simulink model "Motoring_Gear"  (R2024a)
settings: Solver=VariableStepAuto  StartTime=0.0  StopTime=2  FixedStep=1e-6  MaxStep=1e-6  RelTol=1e-6
values from neighbouring files (symbols this model uses):
  B_mod = 0    [Motoring_Gear_param.m]
  Bdc = 1e-4    (= 0.0001)    [Motoring_Gear_param.m]
  BL = 5    [Motoring_Gear_param.m]
  Bs = 1e10    (= 10000000000)    [Motoring_Gear_param.m]
  Bsn = 0    [Motoring_Gear_param.m]
  flux = 0.0563    [Motoring_Gear_param.m]
  J_mod = 5.71e-4    (= 0.000571)    [Motoring_Gear_param.m]
  Jdc = 0.0003    [Motoring_Gear_param.m]
  Jsn = 3.16e-4    (= 0.000316)    [Motoring_Gear_param.m]
  Kag = 0.001    [Motoring_Gear_param.m]
  Kc = 1000000    [Motoring_Gear_param.m]
  Ke = 0.0164    [Motoring_Gear_param.m]
  Kt = 0.0164    [Motoring_Gear_param.m]
  Ld = 3e-5    (= 3e-05)    [Motoring_Gear_param.m]
  Ldc = 8.76e-5    (= 8.76e-05)    [Motoring_Gear_param.m]
  Lq = 3e-5    (= 3e-05)    [Motoring_Gear_param.m]
  Pa = 2    [Motoring_Gear_param.m]
  Psn = 9    [Motoring_Gear_param.m]
  q_mod = 11    [Motoring_Gear_param.m]
  Rs = 0.01    [Motoring_Gear_param.m]
  Rs_dc = 0.01    [Motoring_Gear_param.m]
  velocity_Ki_pi = Bdc*motor_bw    (= 0.0628318530718)    [Motoring_Gear_param.m]
  velocity_Kp_pi = Jdc*motor_bw    (= 0.188495559215)    [Motoring_Gear_param.m]
libraries: cstblocks x2
(part 1 of 2)
settings Model: Creator=User  LastModifiedBy=edlin
settings DebuggingCC: UnconnectedInputMsg=warning  UnconnectedOutputMsg=warning  UnconnectedLineMsg=warning
settings ModelReferenceCC: EnableRefExpFcnMdlSchedulingChecks=on
settings RTWCC: GPUComputeCapability=3.5  DLArmComputeVersion=19.05

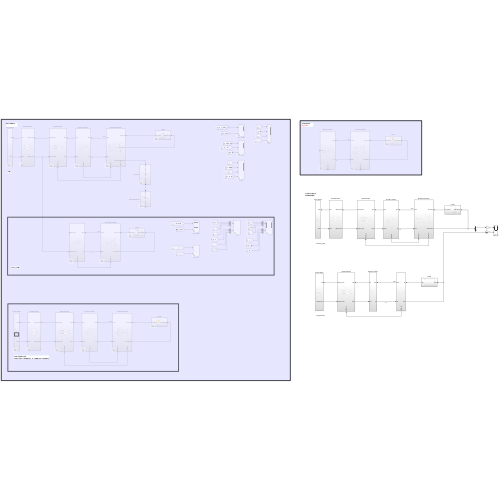
[thumbnail: Simulink's stored preview of the top-level diagram]
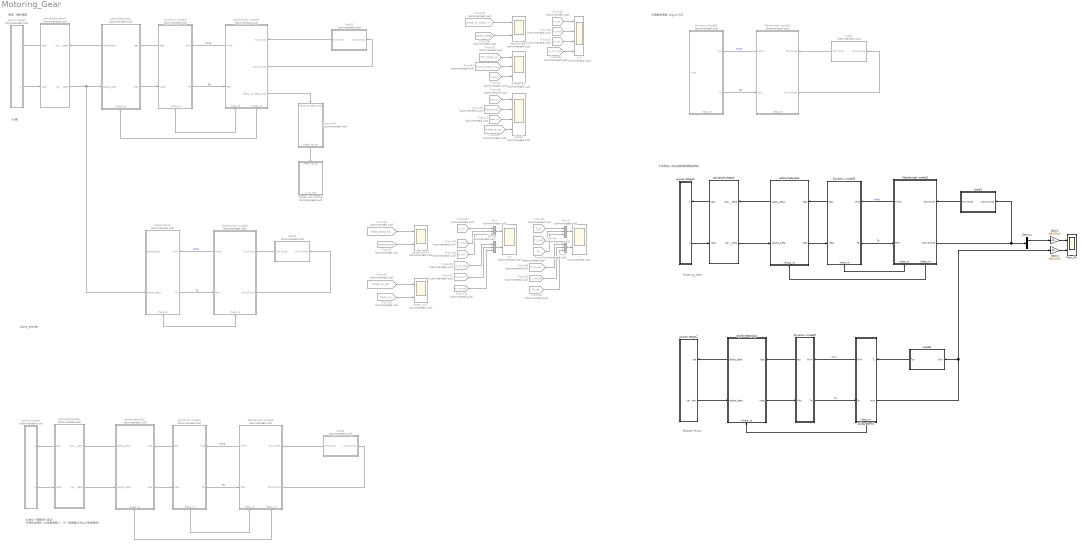
== system Motoring_Gear ==
  note: dq軸=>電壓源打直流
      | 中環或內還其一加負載當輸入，另一個當輸出(BL=0無負載角)
  note: Alpha_beta軸
  note: dq軸
  note: 反電動勢模擬 Kag=0.001
  note: 轉速、轉矩模擬
  note: 步進馬達vs磁性齒輪電機轉速模擬
  note: Motoring_Gear
  note: Stepper Motor
  Demux : Demux  Outputs=2
  Dynamic model1 : Subsystem  Commented=on
      settings: PortSchema="{\"entries\":[{\"content\":{\"sides\":[{\"content\":{\"connectorIds\":[\"In1\"]},\"type\":\"ConnectorPlacement.EquallySpacedRectSide\",\"uuid\":\"7c4d09e5-7ce3-4b20-8435-0def56d6c449\"},{\"content\":{\"connectorIds\":[\"In2\",\"Out1\"],\"side\":\"RIGHT\"},\"type\":\"ConnectorPlacement.EquallySpacedRectSide\",\"uuid\":\"93c63514-3f6b-48a8-aca2-b188521502f4\"},{\"content\":{\"connectorIds\":[],\"side\":\"TOP\"},\"type\":\"ConnectorPlacement.EquallySpacedRectSide\",\"uuid\":\"471dc423-a39c-4f8b-97d0-231d7e49bf1b\"},{\"content\":{\"connectorIds\":[\"Out2\"],\"side\":\"BOTTOM\"},\"type\":\"ConnectorPlacement.EquallySpacedRectSide\",\"uuid\":\"925e2c8f-0b09-4674-959a-18ac97fd648f\"}]},\"type\":\"ConnectorPlacement.EquallySpacedConnector\",\"uuid\":\"0274136e-6574-4791-859e-bbd37aa1b7b6\"}],\"packageUris\":[\"http://schema.mathworks.com/mf0/Connector/R2020b\"],\"version\":\"1.0\"}"
  Dynamic model2 : Subsystem
      settings: PortSchema="{\"entries\":[{\"content\":{\"sides\":[{\"content\":{\"connectorIds\":[\"Out3\",\"In1\"]},\"type\":\"ConnectorPlacement.EquallySpacedRectSide\",\"uuid\":\"7c4d09e5-7ce3-4b20-8435-0def56d6c449\"},{\"content\":{\"connectorIds\":[\"In2\",\"Out1\"],\"side\":\"RIGHT\"},\"type\":\"ConnectorPlacement.EquallySpacedRectSide\",\"uuid\":\"93c63514-3f6b-48a8-aca2-b188521502f4\"},{\"content\":{\"connectorIds\":[],\"side\":\"TOP\"},\"type\":\"ConnectorPlacement.EquallySpacedRectSide\",\"uuid\":\"471dc423-a39c-4f8b-97d0-231d7e49bf1b\"},{\"content\":{\"connectorIds\":[\"Out2\"],\"side\":\"BOTTOM\"},\"type\":\"ConnectorPlacement.EquallySpacedRectSide\",\"uuid\":\"925e2c8f-0b09-4674-959a-18ac97fd648f\"}]},\"type\":\"ConnectorPlacement.EquallySpacedConnector\",\"uuid\":\"0274136e-6574-4791-859e-bbd37aa1b7b6\"}],\"packageUris\":[\"http://schema.mathworks.com/mf0/Connector/R2020b\"],\"version\":\"1.0\"}"
  Dynamic model3 : Subsystem  Commented=on
      settings: PortSchema="{\"entries\":[{\"content\":{\"sides\":[{\"content\":{\"connectorIds\":[\"Out3\",\"In1\"]},\"type\":\"ConnectorPlacement.EquallySpacedRectSide\",\"uuid\":\"7c4d09e5-7ce3-4b20-8435-0def56d6c449\"},{\"content\":{\"connectorIds\":[\"In2\",\"Out1\"],\"side\":\"RIGHT\"},\"type\":\"ConnectorPlacement.EquallySpacedRectSide\",\"uuid\":\"93c63514-3f6b-48a8-aca2-b188521502f4\"},{\"content\":{\"connectorIds\":[],\"side\":\"TOP\"},\"type\":\"ConnectorPlacement.EquallySpacedRectSide\",\"uuid\":\"471dc423-a39c-4f8b-97d0-231d7e49bf1b\"},{\"content\":{\"connectorIds\":[\"Out2\"],\"side\":\"BOTTOM\"},\"type\":\"ConnectorPlacement.EquallySpacedRectSide\",\"uuid\":\"925e2c8f-0b09-4674-959a-18ac97fd648f\"}]},\"type\":\"ConnectorPlacement.EquallySpacedConnector\",\"uuid\":\"0274136e-6574-4791-859e-bbd37aa1b7b6\"}],\"packageUris\":[\"http://schema.mathworks.com/mf0/Connector/R2020b\"],\"version\":\"1.0\"}"
  Dynamic model4 : Subsystem  Commented=on
      settings: PortSchema="{\"entries\":[{\"content\":{\"sides\":[{\"content\":{\"connectorIds\":[\"Out3\",\"In1\"]},\"type\":\"ConnectorPlacement.EquallySpacedRectSide\",\"uuid\":\"7c4d09e5-7ce3-4b20-8435-0def56d6c449\"},{\"content\":{\"connectorIds\":[\"In2\",\"Out1\"],\"side\":\"RIGHT\"},\"type\":\"ConnectorPlacement.EquallySpacedRectSide\",\"uuid\":\"93c63514-3f6b-48a8-aca2-b188521502f4\"},{\"content\":{\"connectorIds\":[],\"side\":\"TOP\"},\"type\":\"ConnectorPlacement.EquallySpacedRectSide\",\"uuid\":\"471dc423-a39c-4f8b-97d0-231d7e49bf1b\"},{\"content\":{\"connectorIds\":[\"Out2\"],\"side\":\"BOTTOM\"},\"type\":\"ConnectorPlacement.EquallySpacedRectSide\",\"uuid\":\"925e2c8f-0b09-4674-959a-18ac97fd648f\"}]},\"type\":\"ConnectorPlacement.EquallySpacedConnector\",\"uuid\":\"0274136e-6574-4791-859e-bbd37aa1b7b6\"}],\"packageUris\":[\"http://schema.mathworks.com/mf0/Connector/R2020b\"],\"version\":\"1.0\"}"
  Dynamic model7 : Subsystem
      settings: PortSchema="{\"entries\":[{\"content\":{\"sides\":[{\"content\":{\"connectorIds\":[\"Out2\",\"In1\"]},\"type\":\"ConnectorPlacement.EquallySpacedRectSide\",\"uuid\":\"2f3a701f-5eea-44d1-b3a7-dbc1fa0e5c0a\"},{\"content\":{\"connectorIds\":[\"In2\",\"Out1\"],\"side\":\"RIGHT\"},\"type\":\"ConnectorPlacement.EquallySpacedRectSide\",\"uuid\":\"f1e2848b-d963-4e60-9d2d-973e23e5c5d3\"},{\"content\":{\"connectorIds\":[],\"side\":\"TOP\"},\"type\":\"ConnectorPlacement.EquallySpacedRectSide\",\"uuid\":\"f63106b5-8217-4120-80d6-773e81ca5be0\"}]},\"type\":\"ConnectorPlacement.EquallySpacedConnector\",\"uuid\":\"f5c5420c-1a40-42b7-b8dc-8ae6d2428c7a\"}],\"packageUris\":[\"http://schema.mathworks.com/mf0/Connector/R2020b\"],\"version\":\"1.0\"}"
  From25 : From  Commented=on  GotoTag=theta_re_theta_rm
  From26 : From  Commented=on  GotoTag=delta_theta  TagVisibility=global
  From27 : From  Commented=on  GotoTag=theta_rm  TagVisibility=global
  From28 : From  Commented=on  GotoTag=w_rm_res  TagVisibility=global
  From29 : From  Commented=on  GotoTag=theta_re_res  TagVisibility=global
  From30 : From  Commented=on  GotoTag=delta_theta_ab  TagVisibility=global
  From31 : From  Commented=on  GotoTag=delta_theta  TagVisibility=global
  From32 : From  Commented=on  GotoTag=theta_rm_ab  TagVisibility=global
  From33 : From  Commented=on  GotoTag=theta_rm  TagVisibility=global
  From34 : From  Commented=on  GotoTag=w_sn_ab  TagVisibility=global
  From35 : From  Commented=on  GotoTag=w_sn  TagVisibility=global
  From36 : From  Commented=on  GotoTag=w_mod  TagVisibility=global
  From37 : From  Commented=on  GotoTag=Psn_theta_sn  TagVisibility=global
  From38 : From  Commented=on  GotoTag=w_rm  TagVisibility=global
  From39 : From  Commented=on  GotoTag=T_sn_ab  TagVisibility=global
  From40 : From  Commented=on  GotoTag=T_sn  TagVisibility=global
  From41 : From  Commented=on  GotoTag=T_mod  TagVisibility=global
  From42 : From  Commented=on  GotoTag=Te  TagVisibility=global
  From43 : From  Commented=on  GotoTag=Pmod_theta_mod  TagVisibility=global
  From44 : From  Commented=on  GotoTag=theta_re  TagVisibility=global
  From45 : From  Commented=on  GotoTag=w_sn  TagVisibility=global
  From46 : From  Commented=on  GotoTag=w_mod  TagVisibility=global
  From47 : From  Commented=on  GotoTag=w_rm  TagVisibility=global
  From48 : From  Commented=on  GotoTag=theta_sn  TagVisibility=global
  From49 : From  Commented=on  GotoTag=theta_mod  TagVisibility=global
  From50 : From  Commented=on  GotoTag=w_rm_ab  TagVisibility=global
  From51 : From  Commented=on  GotoTag=w_mod_ab  TagVisibility=global
  From52 : From  Commented=on  GotoTag=Te_ab  TagVisibility=global
  From53 : From  Commented=on  GotoTag=T_mod_ab  TagVisibility=global
  Gain1 : Gain  Gain=60/(2*pi)
  Gain4 : Gain  Gain=60/(2*pi)
  Load1 : Subsystem  Commented=on
  Load2 : Subsystem
  Load3 : Subsystem  Commented=on
  Load4 : Subsystem  Commented=on
  Load5 : Subsystem  Commented=on
  Load6 : Subsystem
  Mechanical model1 : Subsystem  Commented=on
      settings: PortSchema="{\"entries\":[{\"content\":{\"sides\":[{\"content\":{\"connectorIds\":[\"Out2\",\"In1\"]},\"type\":\"ConnectorPlacement.EquallySpacedRectSide\",\"uuid\":\"27605504-0523-4623-b6f6-c9db4039f2d5\"},{\"content\":{\"connectorIds\":[\"In3\",\"Out1\"],\"side\":\"RIGHT\"},\"type\":\"ConnectorPlacement.EquallySpacedRectSide\",\"uuid\":\"20e727a9-aae7-4835-9463-ae6805ad2222\"},{\"content\":{\"connectorIds\":[],\"side\":\"TOP\"},\"type\":\"ConnectorPlacement.EquallySpacedRectSide\",\"uuid\":\"646511f2-a7bf-4324-af53-134f9ba550e9\"},{\"content\":{\"connectorIds\":[\"In2\"],\"side\":\"BOTTOM\"},\"type\":\"ConnectorPlacement.EquallySpacedRectSide\",\"uuid\":\"7eed8b1f-570c-458f-9984-581d7b55b244\"}]},\"type\":\"ConnectorPlacement.EquallySpacedConnector\",\"uuid\":\"62067768-bb43-41b2-88f6-4544d79748ee\"}],\"packageUris\":[\"http://schema.mathworks.com/mf0/Connector/R2020b\"],\"version\":\"1.0\"}"
  Mechanical model2 : Subsystem
      settings: PortSchema="{\"entries\":[{\"content\":{\"sides\":[{\"content\":{\"connectorIds\":[\"Out3\",\"In1\"]},\"type\":\"ConnectorPlacement.EquallySpacedRectSide\",\"uuid\":\"27605504-0523-4623-b6f6-c9db4039f2d5\"},{\"content\":{\"connectorIds\":[\"In3\",\"Out1\"],\"side\":\"RIGHT\"},\"type\":\"ConnectorPlacement.EquallySpacedRectSide\",\"uuid\":\"20e727a9-aae7-4835-9463-ae6805ad2222\"},{\"content\":{\"connectorIds\":[],\"side\":\"TOP\"},\"type\":\"ConnectorPlacement.EquallySpacedRectSide\",\"uuid\":\"646511f2-a7bf-4324-af53-134f9ba550e9\"},{\"content\":{\"connectorIds\":[\"In2\",\"Out2\"],\"side\":\"BOTTOM\"},\"type\":\"ConnectorPlacement.EquallySpacedRectSide\",\"uuid\":\"7eed8b1f-570c-458f-9984-581d7b55b244\"}]},\"type\":\"ConnectorPlacement.EquallySpacedConnector\",\"uuid\":\"62067768-bb43-41b2-88f6-4544d79748ee\"}],\"packageUris\":[\"http://schema.mathworks.com/mf0/Connector/R2020b\"],\"version\":\"1.0\"}"
  Mechanical model4 : Subsystem  Commented=on
      settings: PortSchema="{\"entries\":[{\"content\":{\"sides\":[{\"content\":{\"connectorIds\":[\"Out3\",\"In1\"]},\"type\":\"ConnectorPlacement.EquallySpacedRectSide\",\"uuid\":\"27605504-0523-4623-b6f6-c9db4039f2d5\"},{\"content\":{\"connectorIds\":[\"In3\",\"Out1\"],\"side\":\"RIGHT\"},\"type\":\"ConnectorPlacement.EquallySpacedRectSide\",\"uuid\":\"20e727a9-aae7-4835-9463-ae6805ad2222\"},{\"content\":{\"connectorIds\":[],\"side\":\"TOP\"},\"type\":\"ConnectorPlacement.EquallySpacedRectSide\",\"uuid\":\"646511f2-a7bf-4324-af53-134f9ba550e9\"},{\"content\":{\"connectorIds\":[\"In2\",\"Out2\"],\"side\":\"BOTTOM\"},\"type\":\"ConnectorPlacement.EquallySpacedRectSide\",\"uuid\":\"7eed8b1f-570c-458f-9984-581d7b55b244\"}]},\"type\":\"ConnectorPlacement.EquallySpacedConnector\",\"uuid\":\"62067768-bb43-41b2-88f6-4544d79748ee\"}],\"packageUris\":[\"http://schema.mathworks.com/mf0/Connector/R2020b\"],\"version\":\"1.0\"}"
  Mechanical model5 : Subsystem  Commented=on
      settings: PortSchema="{\"entries\":[{\"content\":{\"sides\":[{\"content\":{\"connectorIds\":[\"Out4\",\"In1\"]},\"type\":\"ConnectorPlacement.EquallySpacedRectSide\",\"uuid\":\"27605504-0523-4623-b6f6-c9db4039f2d5\"},{\"content\":{\"connectorIds\":[\"In3\",\"Out1\",\"Out2\"],\"side\":\"RIGHT\"},\"type\":\"ConnectorPlacement.EquallySpacedRectSide\",\"uuid\":\"20e727a9-aae7-4835-9463-ae6805ad2222\"},{\"content\":{\"connectorIds\":[],\"side\":\"TOP\"},\"type\":\"ConnectorPlacement.EquallySpacedRectSide\",\"uuid\":\"646511f2-a7bf-4324-af53-134f9ba550e9\"},{\"content\":{\"connectorIds\":[\"In2\",\"Out3\"],\"side\":\"BOTTOM\"},\"type\":\"ConnectorPlacement.EquallySpacedRectSide\",\"uuid\":\"7eed8b1f-570c-458f-9984-581d7b55b244\"}]},\"type\":\"ConnectorPlacement.EquallySpacedConnector\",\"uuid\":\"62067768-bb43-41b2-88f6-4544d79748ee\"}],\"packageUris\":[\"http://schema.mathworks.com/mf0/Connector/R2020b\"],\"version\":\"1.0\"}"
  Mechanical model6 : Subsystem  Commented=on
      settings: PortSchema="{\"entries\":[{\"content\":{\"sides\":[{\"content\":{\"connectorIds\":[\"Out2\",\"In1\"]},\"type\":\"ConnectorPlacement.EquallySpacedRectSide\",\"uuid\":\"27605504-0523-4623-b6f6-c9db4039f2d5\"},{\"content\":{\"connectorIds\":[\"In3\",\"Out1\"],\"side\":\"RIGHT\"},\"type\":\"ConnectorPlacement.EquallySpacedRectSide\",\"uuid\":\"20e727a9-aae7-4835-9463-ae6805ad2222\"},{\"content\":{\"connectorIds\":[],\"side\":\"TOP\"},\"type\":\"ConnectorPlacement.EquallySpacedRectSide\",\"uuid\":\"646511f2-a7bf-4324-af53-134f9ba550e9\"},{\"content\":{\"connectorIds\":[\"In2\"],\"side\":\"BOTTOM\"},\"type\":\"ConnectorPlacement.EquallySpacedRectSide\",\"uuid\":\"7eed8b1f-570c-458f-9984-581d7b55b244\"}]},\"type\":\"ConnectorPlacement.EquallySpacedConnector\",\"uuid\":\"62067768-bb43-41b2-88f6-4544d79748ee\"}],\"packageUris\":[\"http://schema.mathworks.com/mf0/Connector/R2020b\"],\"version\":\"1.0\"}"
  Mux{,1..3} (4 alike) : Mux  Commented=on  Inputs=3
  Speed Estimator2 : Subsystem  Commented=on
  Subsystem2 : Subsystem  Commented=on
      settings: PortSchema="{\"entries\":[{\"content\":{\"sides\":[{\"content\":{\"connectorIds\":[\"Out3\",\"In1\"]},\"type\":\"ConnectorPlacement.EquallySpacedRectSide\",\"uuid\":\"fa0b9505-c3a6-4058-977f-a83052923eff\"},{\"content\":{\"connectorIds\":[\"In2\",\"Out1\"],\"side\":\"RIGHT\"},\"type\":\"ConnectorPlacement.EquallySpacedRectSide\",\"uuid\":\"15c4a0d7-a58e-46bd-a71c-d195b5de468b\"},{\"content\":{\"connectorIds\":[],\"side\":\"TOP\"},\"type\":\"ConnectorPlacement.EquallySpacedRectSide\",\"uuid\":\"1946702f-ff85-49ed-b29f-8291a461de4d\"},{\"content\":{\"connectorIds\":[\"Out2\"],\"side\":\"BOTTOM\"},\"type\":\"ConnectorPlacement.EquallySpacedRectSide\",\"uuid\":\"87d5c706-d909-4315-bee2-4564ae0d4d09\"}]},\"type\":\"ConnectorPlacement.EquallySpacedConnector\",\"uuid\":\"a1672868-2e4d-40bc-a8c0-51f83bb2eeef\"}],\"packageUris\":[\"http://schema.mathworks.com/mf0/Connector/R2020b\"],\"version\":\"1.0\"}"
  Subsystem6 : Subsystem
      settings: PortSchema="{\"entries\":[{\"content\":{\"sides\":[{\"content\":{\"connectorIds\":[\"Out3\",\"In1\"]},\"type\":\"ConnectorPlacement.EquallySpacedRectSide\",\"uuid\":\"680c3f9d-14a9-4663-a7e5-7114b5db478c\"},{\"content\":{\"connectorIds\":[\"In2\",\"Out1\"],\"side\":\"RIGHT\"},\"type\":\"ConnectorPlacement.EquallySpacedRectSide\",\"uuid\":\"ae37b73f-3b71-42af-8a79-21b2839c0d3b\"},{\"content\":{\"connectorIds\":[],\"side\":\"TOP\"},\"type\":\"ConnectorPlacement.EquallySpacedRectSide\",\"uuid\":\"39395bbc-a80a-4c5b-8c9e-521328f6b06f\"},{\"content\":{\"connectorIds\":[\"Out2\"],\"side\":\"BOTTOM\"},\"type\":\"ConnectorPlacement.EquallySpacedRectSide\",\"uuid\":\"0226908e-463a-4058-8ab7-934587d61e58\"}]},\"type\":\"ConnectorPlacement.EquallySpacedConnector\",\"uuid\":\"4732a63d-5c77-40b8-b765-8b8c742822fc\"}],\"packageUris\":[\"http://schema.mathworks.com/mf0/Connector/R2020b\"],\"version\":\"1.0\"}"
  Wsn_Wr : Scope  NumInputPorts=2
  abc/alpha-beta1 : Subsystem
      settings: PortSchema="{\"entries\":[{\"content\":{\"sides\":[{\"content\":{\"connectorIds\":[\"Out2\",\"In1\"]},\"type\":\"ConnectorPlacement.EquallySpacedRectSide\",\"uuid\":\"e35c69ec-9f86-4a67-a4da-903d2966164a\"},{\"content\":{\"connectorIds\":[\"In2\",\"Out1\"],\"side\":\"RIGHT\"},\"type\":\"ConnectorPlacement.EquallySpacedRectSide\",\"uuid\":\"76784336-1844-4d14-a645-4cf1c517120a\"},{\"content\":{\"connectorIds\":[],\"side\":\"TOP\"},\"type\":\"ConnectorPlacement.EquallySpacedRectSide\",\"uuid\":\"124045cf-1007-43ca-a402-978c1e0c157a\"}]},\"type\":\"ConnectorPlacement.EquallySpacedConnector\",\"uuid\":\"8ef95d7c-a81f-46e1-b9bf-f2cf67dc79b8\"}],\"packageUris\":[\"http://schema.mathworks.com/mf0/Connector/R2020b\"],\"version\":\"1.0\"}"
  abc/alpha-beta3 : Subsystem  Commented=on
      settings: PortSchema="{\"entries\":[{\"content\":{\"sides\":[{\"content\":{\"connectorIds\":[\"Out2\",\"In1\"]},\"type\":\"ConnectorPlacement.EquallySpacedRectSide\",\"uuid\":\"e35c69ec-9f86-4a67-a4da-903d2966164a\"},{\"content\":{\"connectorIds\":[\"In2\",\"Out1\"],\"side\":\"RIGHT\"},\"type\":\"ConnectorPlacement.EquallySpacedRectSide\",\"uuid\":\"76784336-1844-4d14-a645-4cf1c517120a\"},{\"content\":{\"connectorIds\":[],\"side\":\"TOP\"},\"type\":\"ConnectorPlacement.EquallySpacedRectSide\",\"uuid\":\"124045cf-1007-43ca-a402-978c1e0c157a\"}]},\"type\":\"ConnectorPlacement.EquallySpacedConnector\",\"uuid\":\"8ef95d7c-a81f-46e1-b9bf-f2cf67dc79b8\"}],\"packageUris\":[\"http://schema.mathworks.com/mf0/Connector/R2020b\"],\"version\":\"1.0\"}"
  abc/alpha-beta4 : Subsystem  Commented=on
      settings: PortSchema="{\"entries\":[{\"content\":{\"sides\":[{\"content\":{\"connectorIds\":[\"Out2\",\"In1\"]},\"type\":\"ConnectorPlacement.EquallySpacedRectSide\",\"uuid\":\"e35c69ec-9f86-4a67-a4da-903d2966164a\"},{\"content\":{\"connectorIds\":[\"In2\",\"Out1\"],\"side\":\"RIGHT\"},\"type\":\"ConnectorPlacement.EquallySpacedRectSide\",\"uuid\":\"76784336-1844-4d14-a645-4cf1c517120a\"},{\"content\":{\"connectorIds\":[],\"side\":\"TOP\"},\"type\":\"ConnectorPlacement.EquallySpacedRectSide\",\"uuid\":\"124045cf-1007-43ca-a402-978c1e0c157a\"}]},\"type\":\"ConnectorPlacement.EquallySpacedConnector\",\"uuid\":\"8ef95d7c-a81f-46e1-b9bf-f2cf67dc79b8\"}],\"packageUris\":[\"http://schema.mathworks.com/mf0/Connector/R2020b\"],\"version\":\"1.0\"}"
  alpha-beta/dq1 : Subsystem
      settings: PortSchema="{\"entries\":[{\"content\":{\"sides\":[{\"content\":{\"connectorIds\":[\"Out2\",\"In1\"]},\"type\":\"ConnectorPlacement.EquallySpacedRectSide\",\"uuid\":\"2b9ad6e5-93b3-42df-bdf3-7a76833e300f\"},{\"content\":{\"connectorIds\":[\"In3\",\"Out1\"],\"side\":\"RIGHT\"},\"type\":\"ConnectorPlacement.EquallySpacedRectSide\",\"uuid\":\"0ae844f9-62d5-4c89-840e-e4e80163c493\"},{\"content\":{\"connectorIds\":[],\"side\":\"TOP\"},\"type\":\"ConnectorPlacement.EquallySpacedRectSide\",\"uuid\":\"b7be56f4-467d-4b7b-a081-48f75f24d7e9\"},{\"content\":{\"connectorIds\":[\"In2\"],\"side\":\"BOTTOM\"},\"type\":\"ConnectorPlacement.EquallySpacedRectSide\",\"uuid\":\"9fd5f3b7-19ba-4245-bc62-f11cca8317c6\"}]},\"type\":\"ConnectorPlacement.EquallySpacedConnector\",\"uuid\":\"d75ca66d-fb38-4ccd-b2dc-598039bc628d\"}],\"packageUris\":[\"http://schema.mathworks.com/mf0/Connector/R2020b\"],\"version\":\"1.0\"}"
  alpha-beta/dq2 : Subsystem  Commented=on
      settings: PortSchema="{\"entries\":[{\"content\":{\"sides\":[{\"content\":{\"connectorIds\":[\"Out2\",\"In1\"]},\"type\":\"ConnectorPlacement.EquallySpacedRectSide\",\"uuid\":\"2b9ad6e5-93b3-42df-bdf3-7a76833e300f\"},{\"content\":{\"connectorIds\":[\"In3\",\"Out1\"],\"side\":\"RIGHT\"},\"type\":\"ConnectorPlacement.EquallySpacedRectSide\",\"uuid\":\"0ae844f9-62d5-4c89-840e-e4e80163c493\"},{\"content\":{\"connectorIds\":[],\"side\":\"TOP\"},\"type\":\"ConnectorPlacement.EquallySpacedRectSide\",\"uuid\":\"b7be56f4-467d-4b7b-a081-48f75f24d7e9\"},{\"content\":{\"connectorIds\":[\"In2\"],\"side\":\"BOTTOM\"},\"type\":\"ConnectorPlacement.EquallySpacedRectSide\",\"uuid\":\"9fd5f3b7-19ba-4245-bc62-f11cca8317c6\"}]},\"type\":\"ConnectorPlacement.EquallySpacedConnector\",\"uuid\":\"d75ca66d-fb38-4ccd-b2dc-598039bc628d\"}],\"packageUris\":[\"http://schema.mathworks.com/mf0/Connector/R2020b\"],\"version\":\"1.0\"}"
  alpha-beta/dq3 : Subsystem  Commented=on
      settings: PortSchema="{\"entries\":[{\"content\":{\"sides\":[{\"content\":{\"connectorIds\":[\"Out2\",\"In1\"]},\"type\":\"ConnectorPlacement.EquallySpacedRectSide\",\"uuid\":\"2b9ad6e5-93b3-42df-bdf3-7a76833e300f\"},{\"content\":{\"connectorIds\":[\"In3\",\"Out1\"],\"side\":\"RIGHT\"},\"type\":\"ConnectorPlacement.EquallySpacedRectSide\",\"uuid\":\"0ae844f9-62d5-4c89-840e-e4e80163c493\"},{\"content\":{\"connectorIds\":[],\"side\":\"TOP\"},\"type\":\"ConnectorPlacement.EquallySpacedRectSide\",\"uuid\":\"b7be56f4-467d-4b7b-a081-48f75f24d7e9\"},{\"content\":{\"connectorIds\":[\"In2\"],\"side\":\"BOTTOM\"},\"type\":\"ConnectorPlacement.EquallySpacedRectSide\",\"uuid\":\"9fd5f3b7-19ba-4245-bc62-f11cca8317c6\"}]},\"type\":\"ConnectorPlacement.EquallySpacedConnector\",\"uuid\":\"d75ca66d-fb38-4ccd-b2dc-598039bc628d\"}],\"packageUris\":[\"http://schema.mathworks.com/mf0/Connector/R2020b\"],\"version\":\"1.0\"}"
  alpha-beta/dq4 : Subsystem
      settings: PortSchema="{\"entries\":[{\"content\":{\"sides\":[{\"content\":{\"connectorIds\":[\"Out2\",\"In1\"]},\"type\":\"ConnectorPlacement.EquallySpacedRectSide\",\"uuid\":\"2b9ad6e5-93b3-42df-bdf3-7a76833e300f\"},{\"content\":{\"connectorIds\":[\"In3\",\"Out1\"],\"side\":\"RIGHT\"},\"type\":\"ConnectorPlacement.EquallySpacedRectSide\",\"uuid\":\"0ae844f9-62d5-4c89-840e-e4e80163c493\"},{\"content\":{\"connectorIds\":[],\"side\":\"TOP\"},\"type\":\"ConnectorPlacement.EquallySpacedRectSide\",\"uuid\":\"b7be56f4-467d-4b7b-a081-48f75f24d7e9\"},{\"content\":{\"connectorIds\":[\"In2\"],\"side\":\"BOTTOM\"},\"type\":\"ConnectorPlacement.EquallySpacedRectSide\",\"uuid\":\"9fd5f3b7-19ba-4245-bc62-f11cca8317c6\"}]},\"type\":\"ConnectorPlacement.EquallySpacedConnector\",\"uuid\":\"d75ca66d-fb38-4ccd-b2dc-598039bc628d\"}],\"packageUris\":[\"http://schema.mathworks.com/mf0/Connector/R2020b\"],\"version\":\"1.0\"}"
  delta_theta2 : Scope  Commented=on  NumInputPorts=2
  delta_theta3 : Scope  Commented=on  NumInputPorts=2
  power stage1 : Subsystem
      settings: PortSchema="{\"entries\":[{\"content\":{\"sides\":[{\"content\":{\"connectorIds\":[]},\"type\":\"ConnectorPlacement.EquallySpacedRectSide\",\"uuid\":\"b8dbbc21-c1f4-4ee6-a4ae-0919678ef684\"},{\"content\":{\"connectorIds\":[\"In1\",\"Out1\"],\"side\":\"RIGHT\"},\"type\":\"ConnectorPlacement.EquallySpacedRectSide\",\"uuid\":\"61e1bbf5-e287-4b89-b804-9623b46ea559\"},{\"content\":{\"connectorIds\":[],\"side\":\"TOP\"},\"type\":\"ConnectorPlacement.EquallySpacedRectSide\",\"uuid\":\"efb7ccb4-1c85-4d0f-b3e5-0bebc17d0910\"}]},\"type\":\"ConnectorPlacement.EquallySpacedConnector\",\"uuid\":\"801d87a2-54d2-4006-a4d4-92ff44eea017\"}],\"packageUris\":[\"http://schema.mathworks.com/mf0/Connector/R2020b\"],\"version\":\"1.0\"}"
  power stage2 : Subsystem
      settings: PortSchema="{\"entries\":[{\"content\":{\"sides\":[{\"content\":{\"connectorIds\":[]},\"type\":\"ConnectorPlacement.EquallySpacedRectSide\",\"uuid\":\"b8dbbc21-c1f4-4ee6-a4ae-0919678ef684\"},{\"content\":{\"connectorIds\":[\"In1\",\"Out1\"],\"side\":\"RIGHT\"},\"type\":\"ConnectorPlacement.EquallySpacedRectSide\",\"uuid\":\"61e1bbf5-e287-4b89-b804-9623b46ea559\"},{\"content\":{\"connectorIds\":[],\"side\":\"TOP\"},\"type\":\"ConnectorPlacement.EquallySpacedRectSide\",\"uuid\":\"efb7ccb4-1c85-4d0f-b3e5-0bebc17d0910\"}]},\"type\":\"ConnectorPlacement.EquallySpacedConnector\",\"uuid\":\"801d87a2-54d2-4006-a4d4-92ff44eea017\"}],\"packageUris\":[\"http://schema.mathworks.com/mf0/Connector/R2020b\"],\"version\":\"1.0\"}"
  power stage3 : Subsystem  Commented=on
      settings: PortSchema="{\"entries\":[{\"content\":{\"sides\":[{\"content\":{\"connectorIds\":[]},\"type\":\"ConnectorPlacement.EquallySpacedRectSide\",\"uuid\":\"b8dbbc21-c1f4-4ee6-a4ae-0919678ef684\"},{\"content\":{\"connectorIds\":[\"In1\",\"Out1\"],\"side\":\"RIGHT\"},\"type\":\"ConnectorPlacement.EquallySpacedRectSide\",\"uuid\":\"61e1bbf5-e287-4b89-b804-9623b46ea559\"},{\"content\":{\"connectorIds\":[],\"side\":\"TOP\"},\"type\":\"ConnectorPlacement.EquallySpacedRectSide\",\"uuid\":\"efb7ccb4-1c85-4d0f-b3e5-0bebc17d0910\"}]},\"type\":\"ConnectorPlacement.EquallySpacedConnector\",\"uuid\":\"801d87a2-54d2-4006-a4d4-92ff44eea017\"}],\"packageUris\":[\"http://schema.mathworks.com/mf0/Connector/R2020b\"],\"version\":\"1.0\"}"
  power stage4 : Subsystem  Commented=on
      settings: PortSchema="{\"entries\":[{\"content\":{\"sides\":[{\"content\":{\"connectorIds\":[]},\"type\":\"ConnectorPlacement.EquallySpacedRectSide\",\"uuid\":\"b8dbbc21-c1f4-4ee6-a4ae-0919678ef684\"},{\"content\":{\"connectorIds\":[\"In1\",\"Out1\"],\"side\":\"RIGHT\"},\"type\":\"ConnectorPlacement.EquallySpacedRectSide\",\"uuid\":\"61e1bbf5-e287-4b89-b804-9623b46ea559\"},{\"content\":{\"connectorIds\":[],\"side\":\"TOP\"},\"type\":\"ConnectorPlacement.EquallySpacedRectSide\",\"uuid\":\"efb7ccb4-1c85-4d0f-b3e5-0bebc17d0910\"}]},\"type\":\"ConnectorPlacement.EquallySpacedConnector\",\"uuid\":\"801d87a2-54d2-4006-a4d4-92ff44eea017\"}],\"packageUris\":[\"http://schema.mathworks.com/mf0/Connector/R2020b\"],\"version\":\"1.0\"}"
  resolver2 : Subsystem  Commented=on
  t : Scope  Commented=on  NumInputPorts=2
  theta1 : Scope  Commented=on  NumInputPorts=4
  theta_re1 : Scope  Commented=on  NumInputPorts=3
  theta_rm1 : Scope  Commented=on  NumInputPorts=2
  w3 : Scope  Commented=on  NumInputPorts=4
  w5 : Scope  Commented=on  NumInputPorts=2
  wires:
  alpha-beta/dq2/1(vdqs) -> Dynamic model3/1(Vdqs)
  abc/alpha-beta3/1(valpha_beta) -> alpha-beta/dq2/1(valpha_beta)
  Mechanical model4/3(*Wre) -> Dynamic model3/2(Wre)  "*Wre"
  alpha-beta/dq2/2(ialpha_beta) -> abc/alpha-beta3/2(ialpha_beta)
  Dynamic model3/2(theta_re) -> Mechanical model4/2(theta_re)
  Mechanical model4/2(*theta_re) -> alpha-beta/dq2/2(*theta_re)
  Dynamic model3/1(Te) -> Mechanical model4/1(Tem)  "Te"
  abc/alpha-beta3/2(iabc) -> power stage3/1(iabc)
  Dynamic model3/3(idqs) -> alpha-beta/dq2/3(idqs)
  Load4/1(Tsn,Tmod) -> Mechanical model4/3(Tsn,Tmod)
  Mechanical model4/1(Wsn,Wmod) -> Load4/1(Wsn,Wmod)
  power stage3/1(vabc) -> abc/alpha-beta3/1(vabc)
  From38/1 -> Mux/3
  From36/1 -> Mux/2
  From35/1 -> Mux/1
  From34/1 -> Mux1/1
  Mechanical model5/2(theta_sn,theta_mod) -> resolver2/1(theta_sn,theta_mod)
  resolver2/1(theta_re_res) -> Speed Estimator2/1(theta_re_res)
  From33/1 -> theta_rm1/2
  From32/1 -> theta_rm1/1
  From30/1 -> delta_theta3/1
  From31/1 -> delta_theta3/2
  Subsystem2/2(theta_re) -> Mechanical model6/2(theta_re)
  Load5/1(Tsn,Tmod) -> Mechanical model6/3(Tsn,Tmod)
  Mechanical model6/1(Wsn,Wmod) -> Load5/1(Wsn,Wmod)
  Subsystem2/1(Te) -> Mechanical model6/1(Tem)  "Te"
  Mechanical model6/2(*Wre) -> Subsystem2/2(Wrm)  "*Wre"
  abc/alpha-beta4/1(valpha_beta) -> Subsystem2/1(Valpha_beta), alpha-beta/dq3/1(valpha_beta)
  From28/1 -> w3/4
  From29/1 -> theta1/4
  From27/1 -> theta1/3
  From49/1 -> theta1/2
  From48/1 -> theta1/1
  From45/1 -> w3/1
  From46/1 -> w3/2
  From47/1 -> w3/3
  From44/1 -> theta_re1/3
  From43/1 -> theta_re1/2
  From37/1 -> theta_re1/1
  From26/1 -> delta_theta2/2
  From25/1 -> delta_theta2/1
  alpha-beta/dq3/1(vdqs) -> Dynamic model4/1(Vdqs)
  Mechanical model5/4(*Wre) -> Dynamic model4/2(Wre)  "*Wre"
  alpha-beta/dq3/2(ialpha_beta) -> abc/alpha-beta4/2(ialpha_beta)
  Dynamic model4/2(theta_re) -> Mechanical model5/2(theta_re)
  power stage4/1(vabc) -> abc/alpha-beta4/1(vabc)
  Mechanical model5/3(*theta_re) -> alpha-beta/dq3/2(*theta_re)
  Dynamic model4/1(Te) -> Mechanical model5/1(Tem)  "Te"
  abc/alpha-beta4/2(iabc) -> power stage4/1(iabc)
  Dynamic model4/3(idqs) -> alpha-beta/dq3/3(idqs)
  Mechanical model5/1(Wsn,Wmod) -> Load3/1(Wsn,Wmod)
  Load3/1(Tsn,Tmod) -> Mechanical model5/3(Tsn,Tmod)
  From51/1 -> Mux1/2
  From50/1 -> Mux1/3
  From52/1 -> Mux3/3
  From53/1 -> Mux3/2
  From39/1 -> Mux3/1
  From41/1 -> Mux2/2
  From42/1 -> Mux2/3
  From40/1 -> Mux2/1
  Mux/1 -> w5/1
  Mux1/1 -> w5/2
  Mux3/1 -> t/2
  Mux2/1 -> t/1
  Dynamic model1/1(Te) -> Mechanical model1/1(Tem)  "Te"
  Mechanical model1/1(Wsn,Wmod) -> Load1/1(Wsn,Wmod)
  Load1/1(Tsn,Tmod) -> Mechanical model1/3(Tsn,Tmod)
  Mechanical model1/2(*Wre) -> Dynamic model1/2(Wre)  "*Wre"
  Load2/1(Tsn,Tmod) -> Mechanical model2/3(Tsn,Tmod)
  Mechanical model2/1(Wsn,Wmod) -> Load2/1(Wsn,Wmod), Demux/1
  Dynamic model2/3(idqs) -> alpha-beta/dq1/3(idqs)
  abc/alpha-beta1/2(iabc) -> power stage1/1(iabc)
  Dynamic model2/1(Te) -> Mechanical model2/1(Tem)  "Te"
  Mechanical model2/2(theta_rm) -> alpha-beta/dq1/2(*theta_re)
  power stage1/1(vabc) -> abc/alpha-beta1/1(vabc)
  Dynamic model2/2(theta_re) -> Mechanical model2/2(theta_re)
  alpha-beta/dq1/2(ialpha_beta) -> abc/alpha-beta1/2(ialpha_beta)
  Mechanical model2/3(*Wre) -> Dynamic model2/2(Wre)  "*Wre"
  alpha-beta/dq1/1(vdqs) -> Dynamic model2/1(Vdqs)
  abc/alpha-beta1/1(valpha_beta) -> alpha-beta/dq1/1(valpha_beta)
  alpha-beta/dq4/2(ialpha_beta) -> power stage2/1(iab)
  Dynamic model7/2(idq) -> alpha-beta/dq4/3(idqs)
  Load6/1(Tsn) -> Subsystem6/2(TL)
  Dynamic model7/1(Te) -> Subsystem6/1(Te)  "Te"
  Subsystem6/2(theta_rm) -> alpha-beta/dq4/2(*theta_re)
  Subsystem6/3(Wrm) -> Dynamic model7/2(Wrm)  "Wrm"
  alpha-beta/dq4/1(vdqs) -> Dynamic model7/1(Vdq)
  power stage2/1(valpha_beta) -> alpha-beta/dq4/1(valpha_beta)
  Subsystem6/1(wsn) -> Gain4/1, Load6/1(Wsn)
  Gain4/1 -> Wsn_Wr/2
  Gain1/1 -> Wsn_Wr/1
  Demux/1 -> Gain1/1

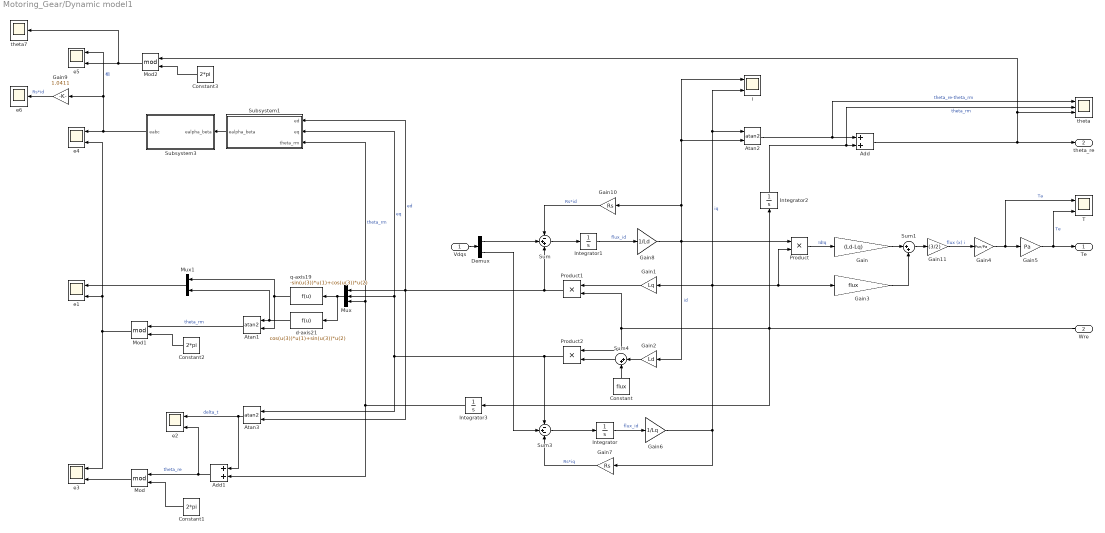
== system Motoring_Gear/Dynamic model1 ==
  Vdqs : Inport
  Wre : Inport  Port=2
  Add : Sum
  Add1 : Sum
  Atan1 : Trigonometry  Operator=atan2
  Atan2 : Trigonometry  Operator=atan2
  Atan3 : Trigonometry  Operator=atan2
  Constant : Constant  Value=flux
  Constant1 : Constant  Value=2*pi
  Constant2 : Constant  Value=2*pi
  Constant3 : Constant  Value=2*pi
  Demux : Demux  Outputs=2
  Gain : Gain  Gain=(Ld-Lq)
  Gain1 : Gain  Gain=Lq
  Gain10 : Gain  Gain=Rs
  Gain11 : Gain  Gain=(3/2)
  Gain2 : Gain  Gain=Ld
  Gain3 : Gain  Gain=flux
  Gain4 : Gain  Gain=Psn/Pa
  Gain5 : Gain  Gain=Pa
  Gain6 : Gain  Gain=1/Lq
  Gain7 : Gain  Gain=Rs
  Gain8 : Gain  Gain=1/Ld
  Gain9 : Gain  Gain=1.0411
  Integrator{,1..3} (4 alike) : Integrator
  Mod : Math  Operator=mod
  Mod1 : Math  Operator=mod
  Mod2 : Math  Operator=mod
  Mux : Mux  Inputs=3
  Mux1 : Mux  Inputs=2
  Product : Product
  Product1 : Product
  Product2 : Product
  Subsystem1 : Subsystem
  Subsystem3 : Subsystem
      settings: PortSchema="{\"entries\":[{\"content\":{\"sides\":[{\"content\":{\"connectorIds\":[\"Out1\"]},\"type\":\"ConnectorPlacement.EquallySpacedRectSide\",\"uuid\":\"b8dbbc21-c1f4-4ee6-a4ae-0919678ef684\"},{\"content\":{\"connectorIds\":[\"In1\"],\"side\":\"RIGHT\"},\"type\":\"ConnectorPlacement.EquallySpacedRectSide\",\"uuid\":\"61e1bbf5-e287-4b89-b804-9623b46ea559\"},{\"content\":{\"connectorIds\":[],\"side\":\"TOP\"},\"type\":\"ConnectorPlacement.EquallySpacedRectSide\",\"uuid\":\"efb7ccb4-1c85-4d0f-b3e5-0bebc17d0910\"}]},\"type\":\"ConnectorPlacement.EquallySpacedConnector\",\"uuid\":\"801d87a2-54d2-4006-a4d4-92ff44eea017\"}],\"packageUris\":[\"http://schema.mathworks.com/mf0/Connector/R2020b\"],\"version\":\"1.0\"}"
  Sum : Sum  Inputs=-++
  Sum1 : Sum  Inputs=|++
  Sum3 : Sum  Inputs=-+-
  Sum4 : Sum  Inputs=|++
  T : Scope  NumInputPorts=2
  d-axis21 : Fcn  Expr=cos(u(3))*u(1)+sin(u(3))*u(2)
  e{1..5} (5 alike) : Scope  NumInputPorts=2
  e6 : Scope
  i : Scope  NumInputPorts=2
  q-axis19 : Fcn  Expr=-sin(u(3))*u(1)+cos(u(3))*u(2)
  theta : Scope  NumInputPorts=3
  theta7 : Scope
  Te : Outport
  theta_re : Outport  Port=2
  wires:
  Gain8/1 -> Gain2/1, i/1, Atan2/2, Gain10/1, Product/1  "id"
  Gain6/1 -> Gain7/1, Gain3/1, Product/2, i/2, Atan2/1, Gain1/1  "iq"
  Add/1 -> theta_re/1, Mod2/1, theta/3
  Integrator/1 -> Gain6/1  "flux_id"
  Integrator1/1 -> Gain8/1  "flux_id"
  Gain4/1 -> Gain5/1, T/1  "Ta"
  Gain11/1 -> Gain4/1  "flux (x) i"
  Gain/1 -> Sum1/1
  Gain1/1 -> Product1/1
  Sum4/1 -> Product2/2
  Constant/1 -> Sum4/2
  Product/1 -> Gain/1  "IdIq"
  Gain2/1 -> Sum4/1
  Gain3/1 -> Sum1/2
  Gain5/1 -> T/2, Te/1  "Te"
  Sum1/1 -> Gain11/1
  Gain7/1 -> Sum3/3  "Rs*iq"
  Demux/2 -> Sum3/2
  Sum3/1 -> Integrator/1
  Sum/1 -> Integrator1/1
  Demux/1 -> Sum/2
  Gain10/1 -> Sum/1  "Rs*id"
  Atan2/1 -> Add/1, theta/1  "theta_re-theta_rm"
  Integrator2/1 -> theta/2, Add/2  "theta_rm"
  Vdqs/1 -> Demux/1
  Mod1/1 -> e3/1, e4/2, e1/2
  Constant2/1 -> Mod1/2
  Constant1/1 -> Mod/2
  q-axis19/1 -> Mux1/1, Atan1/2
  Mod/1 -> e3/2
  Add1/1 -> Mod/1, e2/2  "theta_re"
  Atan3/1 -> Add1/1, e2/1  "delta_t"
  Atan1/1 -> Mod1/1  "theta_rm"
  d-axis21/1 -> Mux1/2, Atan1/1
  Integrator3/1 -> Subsystem1/3(theta_rm), Mux/3, Add1/2  "theta_rm"
  Product2/1 -> Mux/2, Subsystem1/2(eq), Atan3/1, Sum3/1  "eq"
  Mux/1 -> d-axis21/1, q-axis19/1
  Wre/1 -> Product2/1, Product1/2, Integrator3/1, Integrator2/1
  Product1/1 -> Sum/3, Atan3/2, Subsystem1/1(ed), Mux/1  "ed"
  Mux1/1 -> e1/1
  Subsystem1/1(ealpha_beta) -> Subsystem3/1(ealpha_beta)
  Constant3/1 -> Mod2/2
  Subsystem3/1(eabc) -> e5/1, Gain9/1, e4/1  "相"
  Mod2/1 -> theta7/1, e5/2
  Gain9/1 -> e6/1  "Rs*id"

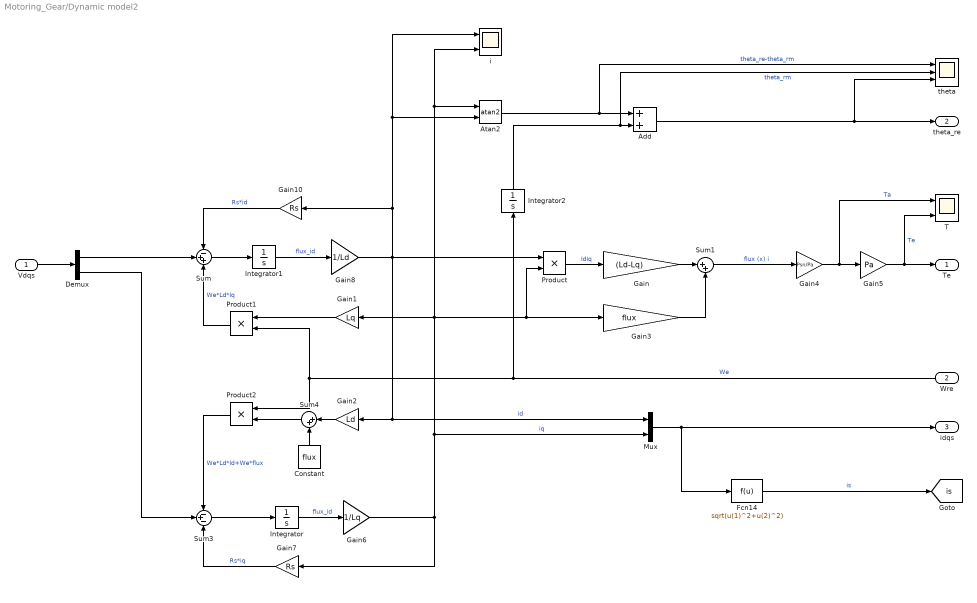
== system Motoring_Gear/Dynamic model2 ==
  Vdqs : Inport
  Wre : Inport  Port=2
  Add : Sum
  Atan2 : Trigonometry  Operator=atan2
  Constant : Constant  Value=flux
  Demux : Demux  Outputs=2
  Fcn14 : Fcn  Expr=sqrt(u(1)^2+u(2)^2)
  Gain : Gain  Gain=(Ld-Lq)
  Gain1 : Gain  Gain=Lq
  Gain10 : Gain  Gain=Rs
  Gain2 : Gain  Gain=Ld
  Gain3 : Gain  Gain=flux
  Gain4 : Gain  Gain=Psn/Pa
  Gain5 : Gain  Gain=Pa
  Gain6 : Gain  Gain=1/Lq
  Gain7 : Gain  Gain=Rs
  Gain8 : Gain  Gain=1/Ld
  Integrator : Integrator
  Integrator1 : Integrator
  Integrator2 : Integrator
  Mux : Mux  Inputs=2
  Product : Product
  Product1 : Product
  Product2 : Product
  Sum : Sum  Inputs=-++
  Sum1 : Sum  Inputs=|++
  Sum3 : Sum  Inputs=-+-
  Sum4 : Sum  Inputs=|++
  T : Scope  NumInputPorts=2
  i : Scope  NumInputPorts=2
  theta : Scope  NumInputPorts=3
  Te : Outport
  theta_re : Outport  Port=2
  idqs : Outport  Port=3
  tag scope: is=global
  wires:
  Gain8/1 -> Gain2/1, Mux/1, i/1, Atan2/2, Gain10/1, Product/1  "id"
  Gain6/1 -> Gain7/1, Gain3/1, Product/2, i/2, Atan2/1, Gain1/1, Mux/2  "iq"
  Add/1 -> theta_re/1, theta/3
  Integrator/1 -> Gain6/1  "flux_id"
  Integrator1/1 -> Gain8/1  "flux_id"
  Gain4/1 -> Gain5/1, T/1  "Ta"
  Sum1/1 -> Gain4/1  "flux (x) i"
  Gain/1 -> Sum1/1
  Product2/1 -> Sum3/1  "We*Ld*Id+We*flux"
  Gain1/1 -> Product1/1
  Wre/1 -> Product2/1, Product1/2, Integrator2/1  "We"
  Sum4/1 -> Product2/2
  Constant/1 -> Sum4/2
  Product1/1 -> Sum/3  "We*Ld*Iq"
  Product/1 -> Gain/1  "IdIq"
  Gain2/1 -> Sum4/1
  Gain3/1 -> Sum1/2
  Gain5/1 -> T/2, Te/1  "Te"
  Gain7/1 -> Sum3/3  "Rs*iq"
  Demux/2 -> Sum3/2
  Sum3/1 -> Integrator/1
  Sum/1 -> Integrator1/1
  Demux/1 -> Sum/2
  Gain10/1 -> Sum/1  "Rs*id"
  Atan2/1 -> Add/1, theta/1  "theta_re-theta_rm"
  Integrator2/1 -> theta/2, Add/2  "theta_rm"
  Vdqs/1 -> Demux/1
  Mux/1 -> Fcn14/1, idqs/1
  Fcn14/1 -> [is]  "is"

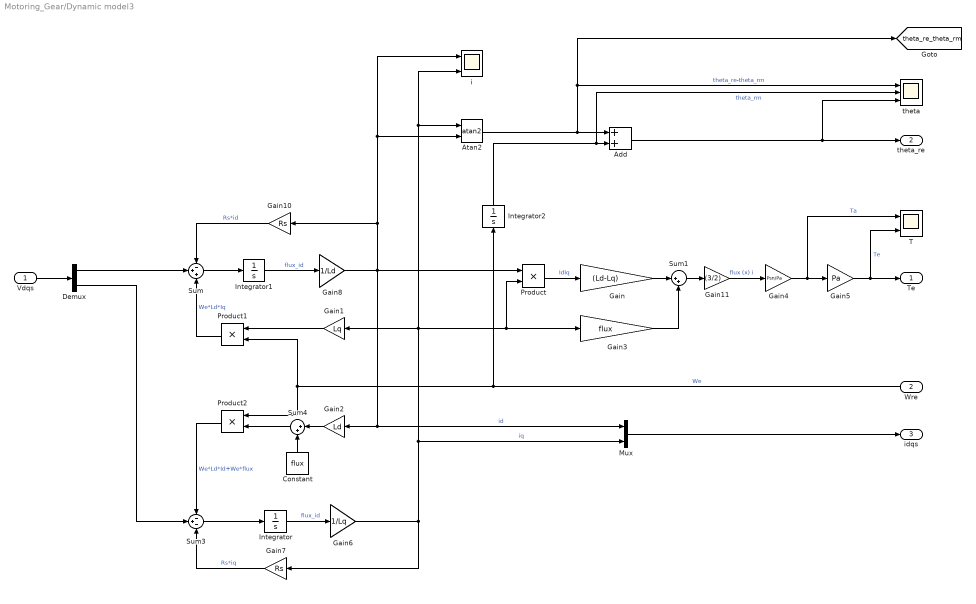
== system Motoring_Gear/Dynamic model3 ==
  Vdqs : Inport
  Wre : Inport  Port=2
  Add : Sum
  Atan2 : Trigonometry  Operator=atan2
  Constant : Constant  Value=flux
  Demux : Demux  Outputs=2
  Gain : Gain  Gain=(Ld-Lq)
  Gain1 : Gain  Gain=Lq
  Gain10 : Gain  Gain=Rs
  Gain11 : Gain  Gain=(3/2)
  Gain2 : Gain  Gain=Ld
  Gain3 : Gain  Gain=flux
  Gain4 : Gain  Gain=Psn/Pa
  Gain5 : Gain  Gain=Pa
  Gain6 : Gain  Gain=1/Lq
  Gain7 : Gain  Gain=Rs
  Gain8 : Gain  Gain=1/Ld
  Integrator : Integrator
  Integrator1 : Integrator
  Integrator2 : Integrator
  Mux : Mux  Inputs=2
  Product : Product
  Product1 : Product
  Product2 : Product
  Sum : Sum  Inputs=-++
  Sum1 : Sum  Inputs=|++
  Sum3 : Sum  Inputs=-+-
  Sum4 : Sum  Inputs=|++
  T : Scope  NumInputPorts=2
  i : Scope  NumInputPorts=2
  theta : Scope  NumInputPorts=3
  Te : Outport
  theta_re : Outport  Port=2
  idqs : Outport  Port=3
  tag scope: theta_re_theta_rm=global
  wires:
  Vdqs/1 -> Demux/1
  Integrator2/1 -> Add/2, theta/2  "theta_rm"
  Atan2/1 -> theta/1, [theta_re_theta_rm], Add/1  "theta_re-theta_rm"
  Gain10/1 -> Sum/1  "Rs*id"
  Demux/1 -> Sum/2
  Sum/1 -> Integrator1/1
  Sum3/1 -> Integrator/1
  Demux/2 -> Sum3/2
  Gain7/1 -> Sum3/3  "Rs*iq"
  Sum1/1 -> Gain11/1
  Gain5/1 -> Te/1, T/2  "Te"
  Gain3/1 -> Sum1/2
  Gain2/1 -> Sum4/1
  Product/1 -> Gain/1  "IdIq"
  Product1/1 -> Sum/3  "We*Ld*Iq"
  Constant/1 -> Sum4/2
  Sum4/1 -> Product2/2
  Wre/1 -> Integrator2/1, Product1/2, Product2/1  "We"
  Gain1/1 -> Product1/1
  Product2/1 -> Sum3/1  "We*Ld*Id+We*flux"
  Gain/1 -> Sum1/1
  Gain11/1 -> Gain4/1  "flux (x) i"
  Gain4/1 -> T/1, Gain5/1  "Ta"
  Integrator1/1 -> Gain8/1  "flux_id"
  Integrator/1 -> Gain6/1  "flux_id"
  Add/1 -> theta/3, theta_re/1
  Gain6/1 -> Mux/2, Gain1/1, Atan2/1, i/2, Product/2, Gain3/1, Gain7/1  "iq"
  Gain8/1 -> Product/1, Gain10/1, Atan2/2, i/1, Mux/1, Gain2/1  "id"
  Mux/1 -> idqs/1

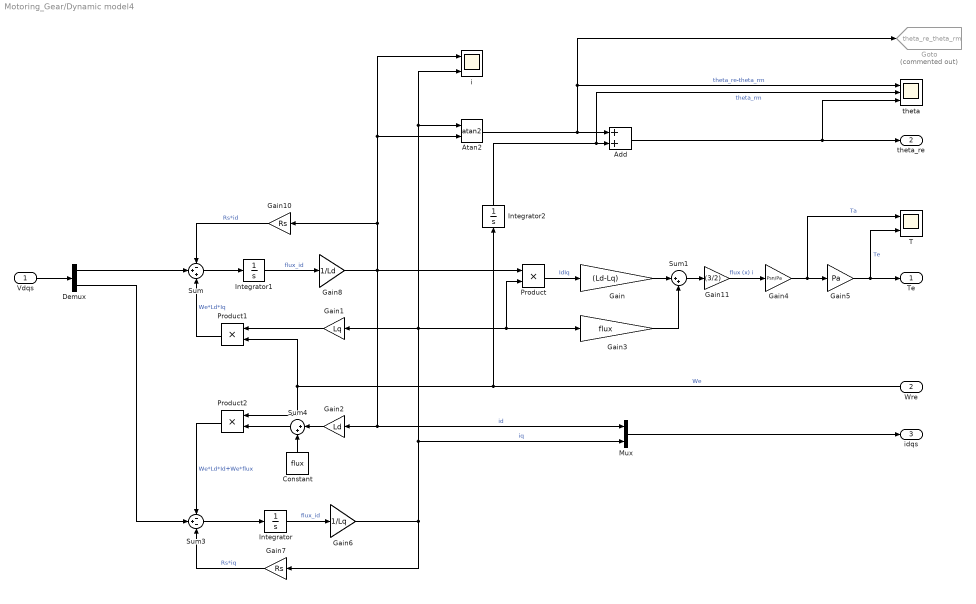
== system Motoring_Gear/Dynamic model4 ==
  Vdqs : Inport
  Wre : Inport  Port=2
  Add : Sum
  Atan2 : Trigonometry  Operator=atan2
  Constant : Constant  Value=flux
  Demux : Demux  Outputs=2
  Gain : Gain  Gain=(Ld-Lq)
  Gain1 : Gain  Gain=Lq
  Gain10 : Gain  Gain=Rs
  Gain11 : Gain  Gain=(3/2)
  Gain2 : Gain  Gain=Ld
  Gain3 : Gain  Gain=flux
  Gain4 : Gain  Gain=Psn/Pa
  Gain5 : Gain  Gain=Pa
  Gain6 : Gain  Gain=1/Lq
  Gain7 : Gain  Gain=Rs
  Gain8 : Gain  Gain=1/Ld
  Goto : Goto  Commented=on  GotoTag=theta_re_theta_rm  TagVisibility=global
  Integrator : Integrator
  Integrator1 : Integrator
  Integrator2 : Integrator
  Mux : Mux  Inputs=2
  Product : Product
  Product1 : Product
  Product2 : Product
  Sum : Sum  Inputs=-++
  Sum1 : Sum  Inputs=|++
  Sum3 : Sum  Inputs=-+-
  Sum4 : Sum  Inputs=|++
  T : Scope  NumInputPorts=2
  i : Scope  NumInputPorts=2
  theta : Scope  NumInputPorts=3
  Te : Outport
  theta_re : Outport  Port=2
  idqs : Outport  Port=3
  wires:
  Vdqs/1 -> Demux/1
  Integrator2/1 -> Add/2, theta/2  "theta_rm"
  Atan2/1 -> theta/1, Goto/1, Add/1  "theta_re-theta_rm"
  Gain10/1 -> Sum/1  "Rs*id"
  Demux/1 -> Sum/2
  Sum/1 -> Integrator1/1
  Sum3/1 -> Integrator/1
  Demux/2 -> Sum3/2
  Gain7/1 -> Sum3/3  "Rs*iq"
  Sum1/1 -> Gain11/1
  Gain5/1 -> Te/1, T/2  "Te"
  Gain3/1 -> Sum1/2
  Gain2/1 -> Sum4/1
  Product/1 -> Gain/1  "IdIq"
  Product1/1 -> Sum/3  "We*Ld*Iq"
  Constant/1 -> Sum4/2
  Sum4/1 -> Product2/2
  Wre/1 -> Integrator2/1, Product1/2, Product2/1  "We"
  Gain1/1 -> Product1/1
  Product2/1 -> Sum3/1  "We*Ld*Id+We*flux"
  Gain/1 -> Sum1/1
  Gain11/1 -> Gain4/1  "flux (x) i"
  Gain4/1 -> T/1, Gain5/1  "Ta"
  Integrator1/1 -> Gain8/1  "flux_id"
  Integrator/1 -> Gain6/1  "flux_id"
  Add/1 -> theta/3, theta_re/1
  Gain6/1 -> Mux/2, Gain1/1, Atan2/1, i/2, Product/2, Gain3/1, Gain7/1  "iq"
  Gain8/1 -> Product/1, Gain10/1, Atan2/2, i/1, Mux/1, Gain2/1  "id"
  Mux/1 -> idqs/1

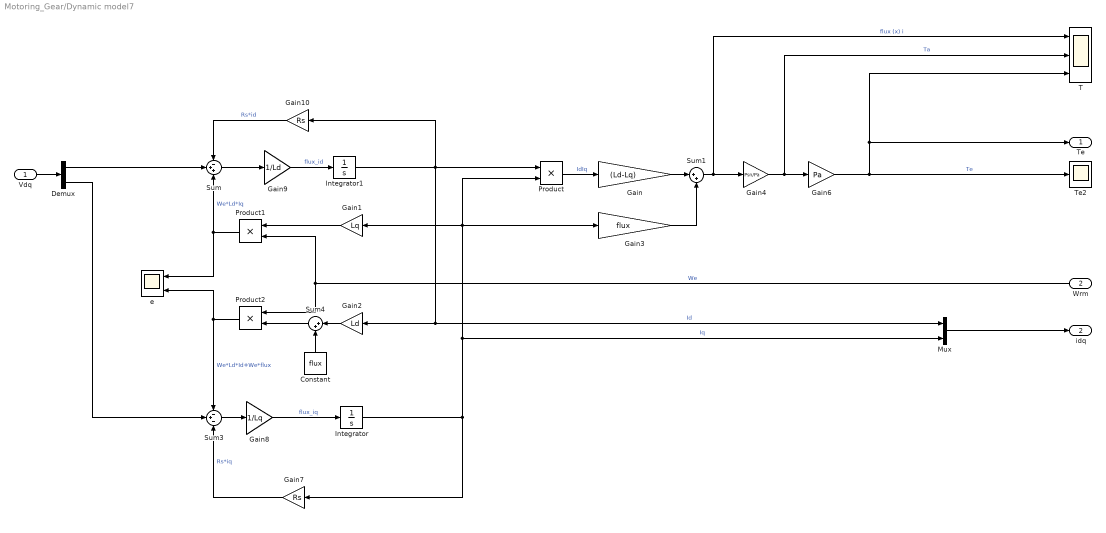
== system Motoring_Gear/Dynamic model7 ==
  Vdq : Inport
  Wrm : Inport  Port=2
  Constant : Constant  Value=flux
  Demux : Demux  Outputs=2
  Gain : Gain  Gain=(Ld-Lq)
  Gain1 : Gain  Gain=Lq
  Gain10 : Gain  Gain=Rs
  Gain2 : Gain  Gain=Ld
  Gain3 : Gain  Gain=flux
  Gain4 : Gain  Gain=Psn/Pa
  Gain6 : Gain  Gain=Pa
  Gain7 : Gain  Gain=Rs
  Gain8 : Gain  Gain=1/Lq
  Gain9 : Gain  Gain=1/Ld
  Integrator : Integrator
  Integrator1 : Integrator
  Mux : Mux  Inputs=2
  Product : Product
  Product1 : Product
  Product2 : Product
  Sum : Sum  Inputs=-++
  Sum1 : Sum  Inputs=|++
  Sum3 : Sum  Inputs=-+-
  Sum4 : Sum  Inputs=|++
  T : Scope  NumInputPorts=3
  Te2 : Scope
  e : Scope  NumInputPorts=2
  Te : Outport
  idq : Outport  Port=2
  wires:
  Gain4/1 -> Gain6/1, T/2  "Ta"
  Gain/1 -> Sum1/1
  Sum/1 -> Gain9/1
  Integrator/1 -> Mux/2, Product/2, Gain3/1, Gain1/1, Gain7/1  "Iq"
  Product2/1 -> Sum3/1, e/2  "We*Ld*Id+We*flux"
  Integrator1/1 -> Mux/1, Gain2/1, Product/1, Gain10/1  "Id"
  Sum3/1 -> Gain8/1
  Gain1/1 -> Product1/1
  Wrm/1 -> Product2/1, Product1/2  "We"
  Sum4/1 -> Product2/2
  Constant/1 -> Sum4/2
  Product1/1 -> Sum/3, e/1  "We*Ld*Iq"
  Product/1 -> Gain/1  "IdIq"
  Gain2/1 -> Sum4/1
  Gain3/1 -> Sum1/2
  Sum1/1 -> Gain4/1, T/1  "flux (x) i"
  Gain7/1 -> Sum3/3  "Rs*iq"
  Demux/2 -> Sum3/2
  Gain8/1 -> Integrator/1  "flux_iq"
  Gain9/1 -> Integrator1/1  "flux_id"
  Demux/1 -> Sum/2
  Gain10/1 -> Sum/1  "Rs*id"
  Gain6/1 -> T/3, Te/1, Te2/1  "Te"
  Vdq/1 -> Demux/1
  Mux/1 -> idq/1

== system Motoring_Gear/Load1 ==
  Wsn,Wmod : Inport
  (2*pi)/60 : Gain  Commented=on  Gain=(2*pi)/60
  DC Motor model(mod) Mod_fixed : Subsystem
      settings: PortSchema="{\"entries\":[{\"content\":{\"sides\":[{\"content\":{\"connectorIds\":[\"In1\"]},\"type\":\"ConnectorPlacement.EquallySpacedRectSide\",\"uuid\":\"2f336b4b-d392-4760-b709-576f7e4aa85b\"},{\"content\":{\"connectorIds\":[],\"side\":\"RIGHT\"},\"type\":\"ConnectorPlacement.EquallySpacedRectSide\",\"uuid\":\"c0607f95-23e7-4738-91c7-666b6347c1d8\"},{\"content\":{\"connectorIds\":[\"Out1\"],\"side\":\"TOP\"},\"type\":\"ConnectorPlacement.EquallySpacedRectSide\",\"uuid\":\"2fb4461d-9d67-45fd-a2c0-63673c9b7e67\"},{\"content\":{\"connectorIds\":[\"In2\"],\"side\":\"BOTTOM\"},\"type\":\"ConnectorPlacement.EquallySpacedRectSide\",\"uuid\":\"2e932aee-a61e-439b-9ee9-2ff1379d0118\"}]},\"type\":\"ConnectorPlacement.EquallySpacedConnector\",\"uuid\":\"170e9b63-2cb1-48dd-b551-4f46129eb95c\"}],\"packageUris\":[\"http://schema.mathworks.com/mf0/Connector/R2020b\"],\"version\":\"1.0\"}"
  DC Motor model(sn) : Subsystem  Commented=on
      settings: PortSchema="{\"entries\":[{\"content\":{\"sides\":[{\"content\":{\"connectorIds\":[\"In1\"]},\"type\":\"ConnectorPlacement.EquallySpacedRectSide\",\"uuid\":\"2f336b4b-d392-4760-b709-576f7e4aa85b\"},{\"content\":{\"connectorIds\":[],\"side\":\"RIGHT\"},\"type\":\"ConnectorPlacement.EquallySpacedRectSide\",\"uuid\":\"c0607f95-23e7-4738-91c7-666b6347c1d8\"},{\"content\":{\"connectorIds\":[\"Out1\"],\"side\":\"TOP\"},\"type\":\"ConnectorPlacement.EquallySpacedRectSide\",\"uuid\":\"2fb4461d-9d67-45fd-a2c0-63673c9b7e67\"},{\"content\":{\"connectorIds\":[\"In2\"],\"side\":\"BOTTOM\"},\"type\":\"ConnectorPlacement.EquallySpacedRectSide\",\"uuid\":\"20971cfd-f73b-4db7-81a1-bf12d69388da\"}]},\"type\":\"ConnectorPlacement.EquallySpacedConnector\",\"uuid\":\"170e9b63-2cb1-48dd-b551-4f46129eb95c\"}],\"packageUris\":[\"http://schema.mathworks.com/mf0/Connector/R2020b\"],\"version\":\"1.0\"}"
  Demux : Demux  Outputs=2
  Gain1 : Gain  Gain=Bs
  Gain21 : Gain  Commented=on  Gain=Bs
  Mux : Mux  Inputs=2
  Step1 : Step  Commented=on  Time=0  Before=100  After=100  SampleTime=0
  Step2 : Step  Time=0  Before=(10*pi)/3  After=(10*pi)/3  SampleTime=0
  Tsn,Tmod : Outport
  wires:
  Mux/1 -> Tsn,Tmod/1
  Wsn,Wmod/1 -> Demux/1
  Demux/1 -> Gain1/1  "Wsn"
  Demux/2 -> DC Motor model(mod) Mod_fixed/2(Wmod)  "Wmod"
  Gain1/1 -> Mux/1
  DC Motor model(mod) Mod_fixed/1(Tmod) -> Mux/2  "Tmod"
  Step1/1 -> (2*pi)/60/1  "Wsn*(rpm)"
  (2*pi)/60/1 -> DC Motor model(sn)/1(Wsn*)  "Wsn*(rad/s)"
  Step2/1 -> DC Motor model(mod) Mod_fixed/1(Wmod*)  "Wmod*"

== system Motoring_Gear/Load2 ==
  Wsn,Wmod : Inport
  Demux : Demux  Outputs=2
  Gain1 : Gain  Gain=BL
  Tsn,Tmod : Outport
  wires:
  Gain1/1 -> Tsn,Tmod/1  "Tsn"
  Wsn,Wmod/1 -> Demux/1
  Demux/1 -> Gain1/1  "Wsn"

== system Motoring_Gear/Load3 ==
  Wsn,Wmod : Inport
  Demux : Demux  Outputs=2
  Gain1 : Gain  Gain=BL
  Gain3 : Gain  Gain=Bs
  Gain4 : Gain  Gain=Bs
  Mux : Mux  Inputs=2
  Scope : Scope  NumInputPorts=2
  Step : Step  Time=0.2  After=0.5  SampleTime=0
  Tsn,Tmod : Outport
  wires:
  Demux/2 -> Gain1/1  "Wmod"
  Demux/1 -> Gain3/1  "Wsn"
  Wsn,Wmod/1 -> Demux/1
  Mux/1 -> Tsn,Tmod/1
  Gain3/1 -> Mux/1
  Gain1/1 -> Mux/2  "Tmod"

== system Motoring_Gear/Load4 ==
  Wsn,Wmod : Inport
  (2*pi)/60 : Gain  Gain=(2*pi)/60
  DC Motor model(mod) Mod_fixed : Subsystem  Commented=on
      settings: PortSchema="{\"entries\":[{\"content\":{\"sides\":[{\"content\":{\"connectorIds\":[\"In1\"]},\"type\":\"ConnectorPlacement.EquallySpacedRectSide\",\"uuid\":\"2f336b4b-d392-4760-b709-576f7e4aa85b\"},{\"content\":{\"connectorIds\":[],\"side\":\"RIGHT\"},\"type\":\"ConnectorPlacement.EquallySpacedRectSide\",\"uuid\":\"c0607f95-23e7-4738-91c7-666b6347c1d8\"},{\"content\":{\"connectorIds\":[\"Out1\"],\"side\":\"TOP\"},\"type\":\"ConnectorPlacement.EquallySpacedRectSide\",\"uuid\":\"2fb4461d-9d67-45fd-a2c0-63673c9b7e67\"},{\"content\":{\"connectorIds\":[\"In2\"],\"side\":\"BOTTOM\"},\"type\":\"ConnectorPlacement.EquallySpacedRectSide\",\"uuid\":\"2e932aee-a61e-439b-9ee9-2ff1379d0118\"}]},\"type\":\"ConnectorPlacement.EquallySpacedConnector\",\"uuid\":\"170e9b63-2cb1-48dd-b551-4f46129eb95c\"}],\"packageUris\":[\"http://schema.mathworks.com/mf0/Connector/R2020b\"],\"version\":\"1.0\"}"
  DC Motor model(sn) : Subsystem
      settings: PortSchema="{\"entries\":[{\"content\":{\"sides\":[{\"content\":{\"connectorIds\":[\"In1\"]},\"type\":\"ConnectorPlacement.EquallySpacedRectSide\",\"uuid\":\"2f336b4b-d392-4760-b709-576f7e4aa85b\"},{\"content\":{\"connectorIds\":[],\"side\":\"RIGHT\"},\"type\":\"ConnectorPlacement.EquallySpacedRectSide\",\"uuid\":\"c0607f95-23e7-4738-91c7-666b6347c1d8\"},{\"content\":{\"connectorIds\":[\"Out1\"],\"side\":\"TOP\"},\"type\":\"ConnectorPlacement.EquallySpacedRectSide\",\"uuid\":\"2fb4461d-9d67-45fd-a2c0-63673c9b7e67\"},{\"content\":{\"connectorIds\":[\"In2\"],\"side\":\"BOTTOM\"},\"type\":\"ConnectorPlacement.EquallySpacedRectSide\",\"uuid\":\"20971cfd-f73b-4db7-81a1-bf12d69388da\"}]},\"type\":\"ConnectorPlacement.EquallySpacedConnector\",\"uuid\":\"170e9b63-2cb1-48dd-b551-4f46129eb95c\"}],\"packageUris\":[\"http://schema.mathworks.com/mf0/Connector/R2020b\"],\"version\":\"1.0\"}"
  Demux : Demux  Outputs=2
  Gain1 : Gain  Commented=on  Gain=Bs
  Gain21 : Gain  Gain=Bs
  Mux : Mux  Inputs=2
  Step1 : Step  Time=0  Before=319  After=319  SampleTime=0
  Step2 : Step  Commented=on  Time=0  Before=(10*pi)/3  After=(10*pi)/3  SampleTime=0
  Step3 : Step  Time=0.2  After=0.5  SampleTime=0
  Tsn,Tmod : Outport
  wires:
  Mux/1 -> Tsn,Tmod/1
  Wsn,Wmod/1 -> Demux/1
  Demux/1 -> DC Motor model(sn)/2(Wsn)  "Wsn"
  Demux/2 -> Gain21/1  "Wmod"
  Step1/1 -> (2*pi)/60/1  "Wsn*(rpm)"
  (2*pi)/60/1 -> DC Motor model(sn)/1(Wsn*)  "Wsn*(rad/s)"
  Step2/1 -> DC Motor model(mod) Mod_fixed/1(Wmod*)  "Wmod*"
  DC Motor model(sn)/1(Tsn) -> Mux/1
  Step3/1 -> Mux/2  "Wsn*(rpm)"

== system Motoring_Gear/Load5 ==
  Wsn,Wmod : Inport
  Demux : Demux  Outputs=2
  Gain20 : Gain  Gain=BL
  Gain21 : Gain  Gain=Bs
  Mux : Mux  Inputs=2
  Tsn,Tmod : Outport
  wires:
  Mux/1 -> Tsn,Tmod/1
  Wsn,Wmod/1 -> Demux/1
  Demux/1 -> Gain20/1  "Wsn"
  Demux/2 -> Gain21/1  "Wmod"
  Gain21/1 -> Mux/2  "Tmod"
  Gain20/1 -> Mux/1

== system Motoring_Gear/Load6 ==
  Wsn : Inport
  Gain21 : Gain  Gain=BL
  Tsn : Outport
  wires:
  Wsn/1 -> Gain21/1  "Wsn"
  Gain21/1 -> Tsn/1

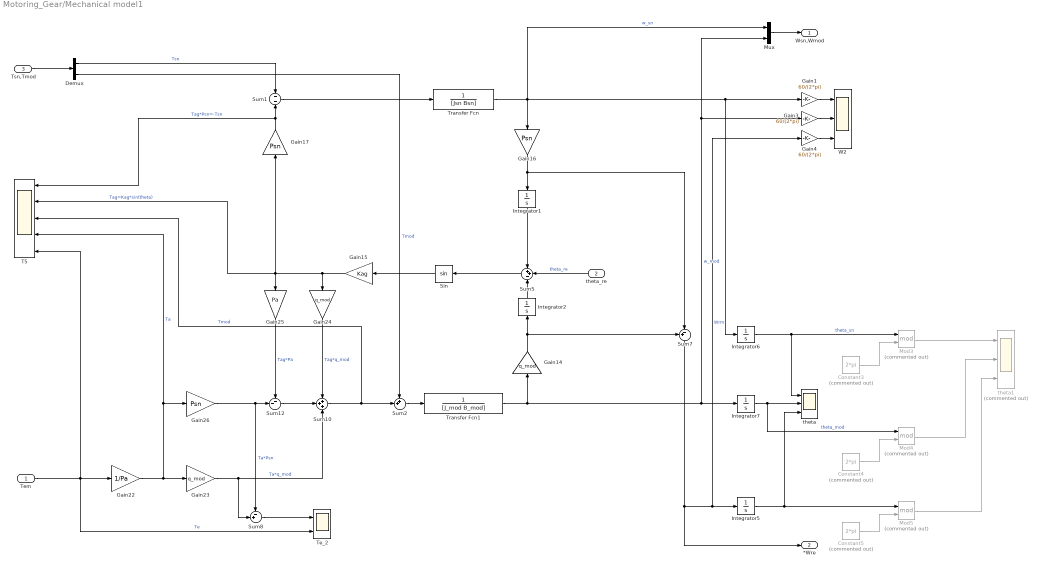
== system Motoring_Gear/Mechanical model1 ==
  Tem : Inport
  theta_re : Inport  Port=2
  Tsn,Tmod : Inport  Port=3
  Constant3 : Constant  Commented=on  Value=2*pi
  Constant4 : Constant  Commented=on  Value=2*pi
  Constant5 : Constant  Commented=on  Value=2*pi
  Demux : Demux  Outputs=2
  Gain1 : Gain  Gain=60/(2*pi)
  Gain14 : Gain  Gain=q_mod
  Gain15 : Gain  Gain=Kag
  Gain16 : Gain  Gain=Psn
  Gain17 : Gain  Gain=Psn
  Gain22 : Gain  Gain=1/Pa
  Gain23 : Gain  Gain=q_mod
  Gain24 : Gain  Gain=q_mod
  Gain25 : Gain  Gain=Pa
  Gain26 : Gain  Gain=Psn
  Gain3 : Gain  Gain=60/(2*pi)
  Gain4 : Gain  Gain=60/(2*pi)
  Integrator{1..2,5..7} (5 alike) : Integrator
  Mod3 : Math  Commented=on  Operator=mod
  Mod4 : Math  Commented=on  Operator=mod
  Mod5 : Math  Commented=on  Operator=mod
  Mux : Mux  Inputs=2
  Sin : Trigonometry
  Sum1 : Sum  Inputs=-|-
  Sum10 : Sum  Inputs=+++
  Sum12 : Sum  Inputs=--|
  Sum2 : Sum  Inputs=++|
  Sum5 : Sum  Inputs=++-
  Sum7 : Sum  Inputs=+-|
  Sum8 : Sum  Inputs=-+|
  T5 : Scope  NumInputPorts=5
  Te_2 : Scope  NumInputPorts=2
  Transfer Fcn : TransferFcn  Denominator=[Jsn Bsn]
  Transfer Fcn1 : TransferFcn  Denominator=[J_mod B_mod]
  W2 : Scope  NumInputPorts=3
  theta : Scope  NumInputPorts=3
  theta1 : Scope  Commented=on  NumInputPorts=3
  Wsn,Wmod : Outport
  *Wre : Outport  Port=2
  wires:
  Demux/2 -> Sum2/1  "Tmod"
  Demux/1 -> Sum1/1  "Tsn"
  Tsn,Tmod/1 -> Demux/1
  Mux/1 -> Wsn,Wmod/1
  Sum8/1 -> Te_2/1
  Transfer Fcn/1 -> Mux/1, Gain16/1, Gain1/1, Integrator6/1  "w_sn"
  Gain17/1 -> T5/1, Sum1/2  "Tag*Psn=-Tsn"
  Gain16/1 -> Integrator1/1, Sum7/2
  Gain15/1 -> Gain25/1, T5/2, Gain17/1, Gain24/1  "Tag=Kag*sin(theta)"
  Sum5/1 -> Sin/1
  Transfer Fcn1/1 -> Gain14/1, Gain3/1, Mux/2, Integrator7/1  "w_mod"
  Tem/1 -> Gain22/1, T5/5, Te_2/2  "Te"
  Sum7/1 -> *Wre/1, Gain4/1, Integrator5/1  "Wrm"
  Gain25/1 -> Sum12/1  "Tag*Pa"
  Gain22/1 -> Gain26/1, T5/4, Gain23/1  "Ta"
  Gain26/1 -> Sum8/1, Sum12/2  "Ta*Psn"
  Sum12/1 -> Sum10/2
  Gain24/1 -> Sum10/1  "Tag*q_mod"
  Gain23/1 -> Sum8/2, Sum10/3  "Ta*q_mod"
  Sum10/1 -> T5/3, Sum2/2  "Tmod"
  Integrator5/1 -> Mod5/1, theta/3
  Integrator6/1 -> theta/1, Mod3/1  "theta_sn"
  Integrator7/1 -> theta/2, Mod4/1  "theta_mod"
  Sin/1 -> Gain15/1
  Sum1/1 -> Transfer Fcn/1
  theta_re/1 -> Sum5/2  "theta_re"
  Sum2/1 -> Transfer Fcn1/1
  Integrator1/1 -> Sum5/1
  Integrator2/1 -> Sum5/3
  Gain14/1 -> Integrator2/1, Sum7/1
  Constant3/1 -> Mod3/2
  Mod3/1 -> theta1/1
  Mod4/1 -> theta1/2
  Constant4/1 -> Mod4/2
  Constant5/1 -> Mod5/2
  Mod5/1 -> theta1/3
  Gain4/1 -> W2/3
  Gain3/1 -> W2/2
  Gain1/1 -> W2/1
